simulink model "simlev"  (R2018a)
settings: Solver=VariableStepAuto  StartTime=0.0  StopTime=10.0  RelTol=1e-3
values from neighbouring files (symbols this model uses):
  A = 2    [sol.m]
  B = 1    [sol.m]
  M = 0.5    [sol.m]
undefined symbols (not defined in the file or in its folder): magnitude
settings Model: Creator=Estudiantes  LastModifiedBy=daniel

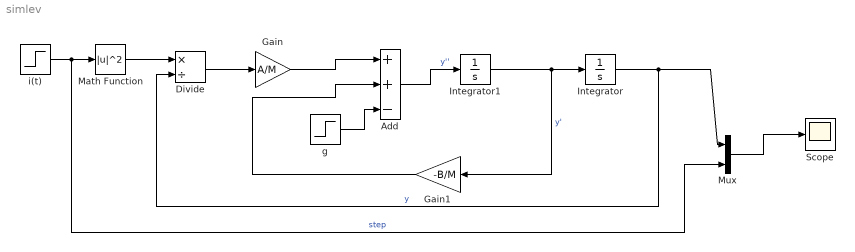
== system simlev ==
  Add : Sum  Inputs=++-
  Divide : Product  Inputs=*/
  Gain : Gain  Gain=A/M
  Gain1 : Gain  Gain=-B/M
  Integrator : Integrator
  Integrator1 : Integrator
  Math Function : Math  Operator=magnitude^2  SaturateOnIntegerOverflow=on
  Mux : Mux  Inputs=2
  Scope : Scope
  "g " : Step  After=9.8  SampleTime=0
  "i(t) " : Step  SampleTime=0
  wires:
  Add/1 -> Integrator1/1  "y''"
  Integrator1/1 -> Gain1/1, Integrator/1  "y'"
  Integrator/1 -> Divide/2, Mux/1  "y"
  Gain1/1 -> Add/2
  Mux/1 -> Scope/1
  "g "/1 -> Add/3
  "i(t) "/1 -> Mux/2, Math Function/1  "step"
  Math Function/1 -> Divide/1
  Divide/1 -> Gain/1
  Gain/1 -> Add/1
